simulink model "MPC_Validation"  (R2020a)
settings: Solver=FixedStepAuto  StartTime=0.0  StopTime=tsim  FixedStep=baseRate  RelTol=1e-3  EnableMultiTasking=on
values from neighbouring files (symbols this model uses):
  Ad = -C(7:12,4:9)    [theFastMPCSolver3.m]    (also in theInitializer.m = dss.A)
  ALGORITHM = 5    [Run_Initializer.m]
  baseRate = 0.05    [Run_Initializer.m]
  cdockdeltax = rc+rt-2*dockoffset    (= 0.165)    [theInitializer.m]
  cdockoa = atan(cdockdeltay/cdockdeltax)    [theInitializer.m]
  Cmat = zeros(6*N,9*N)    [theInitializer.m]
  con0 = [n*N, 2*N, N, N, N]    [Run_Initializer.m]
  drop_states_ARM = [ pi/2, pi/2, 0]    [Run_Initializer.m]
  drop_states_BLACK = rand([1,3])/10+init_states_BLACK    [Run_Initializer.m]
  drop_states_BLUE = rand([1,3])/10+init_states_BLUE    [Run_Initializer.m]
  drop_states_RED = rand([1,3])/10+init_states_RED    [Run_Initializer.m]
  ecoa = pi/2    (= 1.57079632679)    [theInitializer.m]
  F_Black_X_nominal = 0.2196    [Run_Initializer.m]
  F_Black_Y_nominal = 0.2825    [Run_Initializer.m]
  F_Blue_X_nominal = 0.2196    [Run_Initializer.m]
  F_Blue_Y_nominal = 0.2825    [Run_Initializer.m]
  F_red_X_nominal = 0.2196    [Run_Initializer.m]
  F_red_Y_nominal = 0.2825    [Run_Initializer.m]
  F_thrusters_BLACK = [F_Black_X_nominal; F_Black_X_nominal;                             F_Black_Y_nominal; F_Black_Y_nominal; F_Black_X_nominal;                              F_Black_X_nominal; F_Black_Y_nominal; F_Black_Y_nominal]    [Run_Initializer.m]
  F_thrusters_BLUE = [F_Blue_X_nominal; F_Blue_X_nominal;                             F_Blue_Y_nominal; F_Blue_Y_nominal; F_Blue_X_nominal;                              F_Blue_X_nominal; F_Blue_Y_nominal; F_Blue_Y_nominal]    [Run_Initializer.m]
  F_thrusters_RED = [F_red_X_nominal; F_red_X_nominal;                             F_red_Y_nominal; F_red_Y_nominal; F_red_X_nominal;                              F_red_X_nominal; F_red_Y_nominal; F_red_Y_nominal]    [Run_Initializer.m]
  Fmat = reshape(repmat([umax,umax,taumax],N,1),3*N,1)    [theInitializer.m]
  gamma = 0.95    [theInitializer.m]
  Gamma1 = 0.0025    [Run_Initializer.m]
  Gamma2 = 100    [Run_Initializer.m]
  Gamma3 = 10    [Run_Initializer.m]
  Gamma4 = 0.001    [Run_Initializer.m]
  Gamma5 = 100    [Run_Initializer.m]
  Gamma6 = 0.001    [Run_Initializer.m]
  H = blkdiag(pattern{:})    [theInitializer.m]
  home_states_BLACK = [ xLength/2, yLength/2, 0]    [Run_Initializer.m]
  home_states_BLUE = [ xLength/2-0.9, yLength/2+0.5, 0]    [Run_Initializer.m]
  home_states_RED = [ xLength/2+0.7, yLength/2, pi]    [Run_Initializer.m]
  init_states_BLACK = [ct;thetat0].'    [Run_Initializer.m]
  init_states_BLUE = [pobj1;0].'    [Run_Initializer.m]
  init_states_RED = xi(1:3).'    [Run_Initializer.m]
  isCONTROL = 0    [Run_Initializer.m]
  Kd_elarm = 0.05    [Run_Initializer.m]
  Kd_sharm = 0.05    [Run_Initializer.m]
  Kd_tb = 0.4    [Run_Initializer.m]
  Kd_tblue = 0.4    [Run_Initializer.m]
  Kd_tr = 0.4    [Run_Initializer.m]
  Kd_wrarm = 0.005    [Run_Initializer.m]
  Kd_xb = 8    [Run_Initializer.m]
  Kd_xblue = 8    [Run_Initializer.m]
  Kd_xr = 8    [Run_Initializer.m]
  Kd_yb = 8    [Run_Initializer.m]
  Kd_yblue = 8    [Run_Initializer.m]
  Kd_yr = 8    [Run_Initializer.m]
  KOZ_actual = KOZ + rc*sqrt(2)*1.1    [theInitializer.m]
  Kp = [0.08 0 0 ... (first row only)    [Run_Initializer.m]
  Kp_elarm = 0.08    [Run_Initializer.m]
  Kp_sharm = 0.15    [Run_Initializer.m]
  Kp_tb = 0.1    [Run_Initializer.m]
  Kp_tblue = 0.1    [Run_Initializer.m]
  Kp_tr = 0.1    [Run_Initializer.m]
  Kp_wrarm = 0.007    [Run_Initializer.m]
  Kp_xb = 2    [Run_Initializer.m]
  Kp_xblue = 2    [Run_Initializer.m]
  Kp_xr = 2    [Run_Initializer.m]
  Kp_yb = 2    [Run_Initializer.m]
  Kp_yblue = 2    [Run_Initializer.m]
  Kp_yr = 2    [Run_Initializer.m]
  Kv = [0.05 0 0 ... (first row only)    [Run_Initializer.m]
  maxiterations = 10    [Run_Initializer.m]
  N = 15    [Run_Initializer.m]    (also in theFastMPCSolver2.m = length(z)/9; theFastMPCSolver3.m = length(z)/9)
  n = size(b,1)    [my_fbsubstitution.m]    (also in theFastMPCSolver3.m)
  noise_variance_BLACK = 0    [Run_Initializer.m]
  noise_variance_BLUE = 0    [Run_Initializer.m]
  noise_variance_RED = 0    [Run_Initializer.m]
  noisemean = 0.1    [Run_Initializer.m]
  pdockoa = atan(rt/cdockdeltax)    [theInitializer.m]
  pdockr = sqrt(cdockdeltax*cdockdeltax + rt*rt)    [theInitializer.m]
  Phase0_End = Phase0_Duration    (= 5)    [Run_Initializer.m]
  Phase1_End = Phase0_Duration + Phase1_Duration    (= 10)    [Run_Initializer.m]
  Phase2_End = Phase0_Duration + Phase1_Duration +                                   Phase2_Duration    (= 36)    [Run_Initializer.m]
  Phase3_End = Phase0_Duration + Phase1_Duration +                                   Phase2_Duration + Phase3_Duration    (= 166)    [Run_Initializer.m]
  Phase3_SubPhase1_End = Phase2_End + Phase3_SubPhase1_Duration    (= 40)    [Run_Initializer.m]
  Phase3_SubPhase2_End = Phase2_End + Phase3_SubPhase1_Duration +                                   Phase3_SubPhase2_Duration    (= 42)    [Run_Initializer.m]
  Phase3_SubPhase3_End = Phase2_End + Phase3_SubPhase1_Duration +                                   Phase3_SubPhase2_Duration +                                  Phase3_SubPhase3_Duration    (= 44)    [Run_Initializer.m]
  Phase3_SubPhase4_End = Phase2_End + Phase3_SubPhase1_Duration +                                   Phase3_SubPhase2_Duration +                                  Phase3_SubPhase3_Duration +                                  Phase3_SubPhase4_Duration    [Run_Initializer.m]
  Phase4_End = Phase0_Duration + Phase1_Duration +                                   Phase2_Duration + Phase3_Duration +                                   Phase4_Duration    (= 186)    [Run_Initializer.m]
  Phase5_End = Phase0_Duration + Phase1_Duration +                                   Phase2_Duration + Phase3_Duration +                                   Phase4_Duration + Phase5_Duration    (= 191)    [Run_Initializer.m]
  rcone = 0.75    [theInitializer.m]
  rdock = sqrt(cdockdeltax*cdockdeltax + cdockdeltay*cdockdeltay)    [theInitializer.m]
  serverRate = 0.1    [Run_Initializer.m]
  Sj = [KOZ_actual^(-2),0; 0,KOZ_actual^(-2)]    [theInitializer.m]
  taumax = umax*rc    (= 0.0225)    [theInitializer.m]
  Td = 2    [Run_Initializer.m]
  thetah = 20.0 * d2r    (= 0.349065850399)    [theInitializer.m]
  thetat_dot = 0 * d2r    (= 0)    [Run_Initializer.m]
  thruster_dist2CG_BLACK = [83.42;-52.58;55.94;-60.05;54.08;-53.92;77.06;-55.94]    [Run_Initializer.m]
  thruster_dist2CG_BLUE = [73.54;-64.46;81.39;-60.11;64.46;-65.94;54.61;-74.39]    [Run_Initializer.m]
  thruster_dist2CG_RED = [49.92;-78.08;70.46;-63.54;81.08;-50.42;57.44;-75.96]    [Run_Initializer.m]
  tol = 0.00015    [Run_Initializer.m]
  Tz_lim_elarm = .1    (= 0.1)    [Run_Initializer.m]
  Tz_lim_sharm = .1    (= 0.1)    [Run_Initializer.m]
  Tz_lim_wrarm = .1    (= 0.1)    [Run_Initializer.m]
  Umat = zeros(3*N,9*N)    [theInitializer.m]
  umax = 0.15    [theInitializer.m]
  vobj1 = [0.00;0.00]    [Run_Initializer.m]
  vtar = [0.0;0.0]    [Run_Initializer.m]
undefined symbols (not defined in the file or in its folder): DiscIntNeverNeededParam, model_param, platformSelection, simMode, WhoAmI
libraries: dspstat3 x23, dspsigops x15, embdlinuxlib x10, raspberrypiBasiclib x10, simulink x8, MainLibrary x7, mspfiltlib x3, dsparch4 x3, dspswit3 x2, sensehatlib x1
(part 4 of 18)

== system MPC_Validation/Phase #5: Hold Home/Change BLUE Behavior ==
  note: PD Control Law - WHITE
  note: Additional blocks are stored here.
  note: A simple PD control law is used here to command the platform to it's initial position, as defined in the initializer.
  note: Additional Blocks
  Action Port : ActionPort  ActionPortLabel=if(u1 == 3 | u2 == 1)
  BLUE_Fx : DataStoreWrite  DataStoreName=BLUE_Fx
  BLUE_Fy : DataStoreWrite  DataStoreName=BLUE_Fy
  BLUE_Px : DataStoreRead  DataStoreName=BLUE_Px
  "BLUE_Py " : DataStoreRead  DataStoreName=BLUE_Py
  BLUE_Rz : DataStoreRead  DataStoreName=BLUE_Rz
  BLUE_Tz : DataStoreWrite  DataStoreName=BLUE_Tz
  Custom Discrete PD (Attitude) : Subsystem
  Custom Discrete PD (X-Position) : Subsystem
  Custom Discrete PD (Y-Position) : Subsystem
  Data Store Write3 : DataStoreWrite  DataStoreName=Float_State
  Desired Attitude (BLUE) : Constant  Value=home_states_BLUE(3)  SampleTime=-1
  Desired Px (BLUE) : Constant  Value=home_states_BLUE(1)  SampleTime=-1
  Desired Py (BLUE) : Constant  Value=home_states_BLUE(2)  SampleTime=-1
  Hough Control : Subsystem
  Puck State : Constant
  Subtract : Sum  Inputs=+-
  Subtract1 : Sum  Inputs=+-
  wires:
  Puck State/1 -> Data Store Write3/1
  Custom Discrete PD (Y-Position)/1(Fy) -> BLUE_Fy/1
  Custom Discrete PD (X-Position)/1(Fx) -> BLUE_Fx/1
  Subtract1/1 -> Custom Discrete PD (Y-Position)/1(ey)
  "BLUE_Py "/1 -> Subtract1/2
  Desired Px (BLUE)/1 -> Subtract/1
  Hough Control/1(Err) -> Custom Discrete PD (Attitude)/1(ez)
  Subtract/1 -> Custom Discrete PD (X-Position)/1(ex)
  Custom Discrete PD (Attitude)/1(Tz) -> BLUE_Tz/1
  BLUE_Rz/1 -> Hough Control/2(Act)
  Desired Py (BLUE)/1 -> Subtract1/1
  BLUE_Px/1 -> Subtract/2
  Desired Attitude (BLUE)/1 -> Hough Control/1(Ref)

== system MPC_Validation/Phase #5: Hold Home/Change RED Behavior ==
  note: PD Control Law - RED
  note: Additional Blocks
  note: Additional blocks are stored above. Note that to control attitude using the RW, simply replace RED_Tz with RED_Tz_RW.
  note: A simple PD control law is used here to command the platform to it's home position, as defined in the initializer.
  note: ARM Control Law - RED
  Action Port : ActionPort  ActionPortLabel=if(u1 == 1 | u2 == 1)
  Constant1 : Constant  Value=0
  Constant3 : Constant  Value=platformSelection
  Custom Discrete PD (Attitude) : Subsystem
  Custom Discrete PD (X-Position) : Subsystem
  Custom Discrete PD (Y-Position) : Subsystem
  Data Store Write1 : DataStoreWrite  DataStoreName=MPC_State
  Data Store Write3 : DataStoreWrite  DataStoreName=Float_State
  Data Store Write4 : DataStoreWrite  DataStoreName=MPC_State
  Desired Px (BLACK) : Constant  Value=home_states_RED(1)  SampleTime=-1
  Desired Px (BLACK)1 : Constant  Value=home_states_RED(2)  SampleTime=-1
  Desired Px (BLACK)2 : Constant  Value=home_states_RED(3)  SampleTime=-1
  Hough Control : Subsystem
  If : If  IfExpression=u1 == 4 | u1 == 5 | u1 == 10 | u1 == 11
  MPC State : Constant  Value=0
  MPC State1 : Constant  Value=0
  Puck State : Constant
  RED : Subsystem  TreatAsAtomicUnit=on
  RED+ARM : Subsystem  TreatAsAtomicUnit=on
  RED_Fx : DataStoreWrite  DataStoreName=RED_Fx
  RED_Fy : DataStoreWrite  DataStoreName=RED_Fy
  RED_Px : DataStoreRead  DataStoreName=RED_Px
  "RED_Py " : DataStoreRead  DataStoreName=RED_Py
  RED_Rz : DataStoreRead  DataStoreName=RED_Rz
  RED_Tz : DataStoreWrite  DataStoreName=RED_Tz
  RED_Tz_RW : DataStoreWrite  DataStoreName=RED_Tz_RW
  Subtract : Sum  Inputs=+-
  Subtract1 : Sum  Inputs=+-
  wires:
  Constant1/1 -> RED_Tz_RW/1
  Puck State/1 -> Data Store Write3/1
  Desired Px (BLACK)1/1 -> Subtract1/1
  Custom Discrete PD (Attitude)/1(Tz) -> RED_Tz/1
  "RED_Py "/1 -> Subtract1/2
  RED_Rz/1 -> Hough Control/2(Act)
  Desired Px (BLACK)/1 -> Subtract/1
  Custom Discrete PD (Y-Position)/1(Fy) -> RED_Fy/1
  Subtract1/1 -> Custom Discrete PD (Y-Position)/1(ey)
  Custom Discrete PD (X-Position)/1(Fx) -> RED_Fx/1
  Subtract/1 -> Custom Discrete PD (X-Position)/1(ex)
  Hough Control/1(Err) -> Custom Discrete PD (Attitude)/1(ez)
  Desired Px (BLACK)2/1 -> Hough Control/1(Ref)
  RED_Px/1 -> Subtract/2
  If/1 -> RED+ARM/Action
  If/2 -> RED/Action
  Constant3/1 -> If/1
  MPC State/1 -> Data Store Write4/1
  MPC State1/1 -> Data Store Write1/1

== system MPC_Validation/Phase #5: Hold Home/Is this a simulation? ==
  Constant : Constant  Value=simMode  SampleTime=-1
  isSim : Outport  VectorParamsAs1DForOutWhenUnconnected=off
  wires:
  Constant/1 -> isSim/1

== system MPC_Validation/Phase #6: Stop Floating and Spin Down RW/Change BLACK Behavior ==
  note: At the end of the experiment, the pucks must be turned off.
  note: At the end of the experiment, all thrust and arms movement must cease.
  Action Port : ActionPort  ActionPortLabel=if(u1 == 2 | u2 == 1)
  BLACK_Fx : DataStoreWrite  DataStoreName=BLACK_Fx
  BLACK_Fy : DataStoreWrite  DataStoreName=BLACK_Fy
  BLACK_Tz : DataStoreWrite  DataStoreName=BLACK_Tz
  Constant3 : Constant  Value=0
  Constant4 : Constant  Value=0
  Constant5 : Constant  Value=0
  Data Store Write3 : DataStoreWrite  DataStoreName=Float_State
  Puck State : Constant  Value=0
  wires:
  Constant3/1 -> BLACK_Fx/1
  Constant5/1 -> BLACK_Tz/1
  Constant4/1 -> BLACK_Fy/1
  Puck State/1 -> Data Store Write3/1

== system MPC_Validation/Phase #6: Stop Floating and Spin Down RW/Change BLUE Behavior ==
  note: Before getting good data, the platforms must NOT be floating. So, float is set to be "off".
  note: For the initialization phase, we do not want any thrust. Thus, all commanded forces are zero.
  Action Port : ActionPort  ActionPortLabel=if(u1 == 3 | u2 == 1)
  BLUE_Fx : DataStoreWrite  DataStoreName=BLUE_Fx
  BLUE_Fy : DataStoreWrite  DataStoreName=BLUE_Fy
  BLUE_Tz : DataStoreWrite  DataStoreName=BLUE_Tz
  Constant3 : Constant  Value=0
  Constant4 : Constant  Value=0
  Constant5 : Constant  Value=0
  Data Store Write4 : DataStoreWrite  DataStoreName=Float_State
  Puck State : Constant  Value=0
  wires:
  Constant3/1 -> BLUE_Fx/1
  Constant5/1 -> BLUE_Tz/1
  Constant4/1 -> BLUE_Fy/1
  Puck State/1 -> Data Store Write4/1

== system MPC_Validation/Phase #6: Stop Floating and Spin Down RW/Change RED Behavior ==
  note: At the end of the experiment, the pucks must be turned off.
  note: At the end of the experiment, all thrust and arms movement must cease.
  note: Once the platform has settled, the RW must be slowly desaturated (assuming it has been used).
  Action Port : ActionPort  ActionPortLabel=if(u1 == 1 | u2 == 1)
  Constant{,1..2,4..6} (6 alike) : Constant  Value=0
  Data Store Write : DataStoreWrite  DataStoreName=RED_Tz_Shoulder
  Data Store Write1 : DataStoreWrite  DataStoreName=RED_Tz_Elbow
  Data Store Write2 : DataStoreWrite  DataStoreName=RED_Tz_Wrist
  Data Store Write3 : DataStoreWrite  DataStoreName=Float_State
  Data Store Write4 : DataStoreWrite  DataStoreName=MPC_State
  Gain : Gain  Gain=-1
  MPC State : Constant  Value=0
  Puck State : Constant  Value=0
  RED_Fx : DataStoreWrite  DataStoreName=RED_Fx
  RED_Fy : DataStoreWrite  DataStoreName=RED_Fy
  RED_Tz : DataStoreWrite  DataStoreName=RED_Tz
  RED_Tz_RW : DataStoreWrite  DataStoreName=RED_Tz_RW
  RED_dRz_Speed : DataStoreRead  DataStoreName=RED_dRz_RW_Sat
  Saturation : Saturate  UpperLimit=0.005  LowerLimit=-0.005
  wires:
  Constant/1 -> RED_Fx/1
  Constant6/1 -> Data Store Write2/1
  Constant5/1 -> Data Store Write1/1
  RED_dRz_Speed/1 -> Gain/1
  Constant4/1 -> Data Store Write/1
  Saturation/1 -> RED_Tz_RW/1
  Constant1/1 -> RED_Fy/1
  Gain/1 -> Saturation/1
  Constant2/1 -> RED_Tz/1
  Puck State/1 -> Data Store Write3/1
  MPC State/1 -> Data Store Write4/1

== system MPC_Validation/Phase #6: Stop Floating and Spin Down RW/Is this a simulation? ==
  Constant : Constant  Value=simMode  SampleTime=-1
  isSim : Outport  VectorParamsAs1DForOutWhenUnconnected=off
  wires:
  Constant/1 -> isSim/1

== system MPC_Validation/Simulate Plant Dynamics/BLACK Dynamics ==
  note: Above is the dynamic model for the BLACK platform.
  BLACK Dynamics Model : Subsystem  SystemSampleTime=serverRate
  BLACK_Fx_Sat : DataStoreRead  DataStoreName=BLACK_Fx_Sat
  BLACK_Fy_Sat : DataStoreRead  DataStoreName=BLACK_Fy_Sat
  BLACK_IMU_Ax_I : DataStoreWrite  DataStoreName=BLACK_IMU_Ax_I
  BLACK_IMU_Ay_I : DataStoreWrite  DataStoreName=BLACK_IMU_Ay_I
  BLACK_IMU_R : DataStoreWrite  DataStoreName=BLACK_IMU_R
  BLACK_Px : DataStoreWrite  DataStoreName=BLACK_Px
  BLACK_Py : DataStoreWrite  DataStoreName=BLACK_Py
  BLACK_Rz : DataStoreWrite  DataStoreName=BLACK_Rz
  BLACK_RzD : DataStoreWrite  DataStoreName=BLACK_RzD
  BLACK_Tz_Sat : DataStoreRead  DataStoreName=BLACK_Tz_Sat
  BLACK_Vx : DataStoreWrite  DataStoreName=BLACK_Vx
  BLACK_Vy : DataStoreWrite  DataStoreName=BLACK_Vy
  Demux1 : Demux  Outputs=3
  Demux2 : Demux  Outputs=3
  Mux1 : Mux  Inputs=3
  Random Number : RandomNumber  Mean=noisemean  Variance=1.5e-6
  Random Number1 : RandomNumber  Mean=noisemean  Variance=1.5e-6
  Random Number2 : RandomNumber  Mean=noisemean  Variance=1.5e-6
  Sample and Hold Data to Match PhaseSpace (BLACK) : Subsystem
  Sum1 : Sum  Inputs=|++
  Sum2 : Sum  Inputs=|++
  Sum3 : Sum  Inputs=|++
  "x_dot -> x13" : Subsystem
  "x_dot -> x14" : Subsystem
  "x_dot -> x4" : Subsystem
  "x_dot -> x5" : Subsystem
  "x_dot -> x6" : Subsystem
  wires:
  BLACK_Fy_Sat/1 -> Mux1/2
  BLACK_Tz_Sat/1 -> Mux1/3
  Demux1/1 -> BLACK_Px/1
  "x_dot -> x4"/1(dy(t)/dt) -> "x_dot -> x13"/1(y(t)), BLACK_Vx/1
  "x_dot -> x6"/1(dy(t)/dt) -> Sum3/1, BLACK_RzD/1
  Demux1/2 -> BLACK_Py/1
  "x_dot -> x5"/1(dy(t)/dt) -> "x_dot -> x14"/1(y(t)), BLACK_Vy/1
  BLACK_Fx_Sat/1 -> Mux1/1
  Demux2/2 -> "x_dot -> x5"/1(y(t))
  Mux1/1 -> BLACK Dynamics Model/1(control_inputs)
  Demux2/3 -> "x_dot -> x6"/1(y(t))
  Demux1/3 -> BLACK_Rz/1
  Sum3/1 -> BLACK_IMU_R/1
  BLACK Dynamics Model/1(states) -> Sample and Hold Data to Match PhaseSpace (BLACK)/1(states)
  Demux2/1 -> "x_dot -> x4"/1(y(t))
  Sample and Hold Data to Match PhaseSpace (BLACK)/1(states_hold) -> Demux2/1, Demux1/1
  Sum1/1 -> BLACK_IMU_Ax_I/1
  "x_dot -> x13"/1(dy(t)/dt) -> Sum1/1
  Sum2/1 -> BLACK_IMU_Ay_I/1
  Random Number/1 -> Sum2/2
  Random Number2/1 -> Sum3/2
  Random Number1/1 -> Sum1/2
  "x_dot -> x14"/1(dy(t)/dt) -> Sum2/1

== system MPC_Validation/Simulate Plant Dynamics/BLUE Dynamics ==
  note: Above is the dynamic model for the BLUE platform.
  BLUE  Dynamics Model : Subsystem  SystemSampleTime=serverRate
  "BLUE_Fx_Sat " : DataStoreRead  DataStoreName=BLUE_Fx_Sat
  BLUE_Fy_Sat : DataStoreRead  DataStoreName=BLUE_Fy_Sat
  BLUE_IMU_Ax_I : DataStoreWrite  DataStoreName=BLUE_IMU_Ax_I
  BLUE_IMU_Ay_I : DataStoreWrite  DataStoreName=BLUE_IMU_Ay_I
  BLUE_IMU_R : DataStoreWrite  DataStoreName=BLUE_IMU_R
  "BLUE_Px " : DataStoreWrite  DataStoreName=BLUE_Px
  BLUE_Py : DataStoreWrite  DataStoreName=BLUE_Py
  BLUE_Rz : DataStoreWrite  DataStoreName=BLUE_Rz
  BLUE_RzD : DataStoreWrite  DataStoreName=BLUE_RzD
  BLUE_Tz_Sat : DataStoreRead  DataStoreName=BLUE_Tz_Sat
  BLUE_Vx : DataStoreWrite  DataStoreName=BLUE_Vx
  BLUE_Vy : DataStoreWrite  DataStoreName=BLUE_Vy
  Demux4 : Demux  Outputs=3
  Demux5 : Demux  Outputs=3
  Mux2 : Mux  Inputs=3
  Random Number3 : RandomNumber  Mean=noisemean  Variance=1.5e-6
  Random Number4 : RandomNumber  Mean=noisemean  Variance=1.5e-6
  Random Number5 : RandomNumber  Variance=1.5e-6
  Sample and Hold Data to Match PhaseSpace (BLUE) : Subsystem
  Sum4 : Sum  Inputs=|++
  Sum5 : Sum  Inputs=|++
  Sum6 : Sum  Inputs=|++
  "x_dot -> x16" : Subsystem
  "x_dot -> x17" : Subsystem
  "x_dot -> x7" : Subsystem
  "x_dot -> x8" : Subsystem
  "x_dot -> x9" : Subsystem
  wires:
  Sample and Hold Data to Match PhaseSpace (BLUE)/1(states_hold) -> Demux5/1, Demux4/1
  Demux5/3 -> "x_dot -> x9"/1(y(t))
  Demux4/1 -> "BLUE_Px "/1
  Demux4/2 -> BLUE_Py/1
  "BLUE_Fx_Sat "/1 -> Mux2/1
  BLUE_Fy_Sat/1 -> Mux2/2
  Demux5/1 -> "x_dot -> x7"/1(y(t))
  BLUE_Tz_Sat/1 -> Mux2/3
  Demux4/3 -> BLUE_Rz/1
  BLUE  Dynamics Model/1(states) -> Sample and Hold Data to Match PhaseSpace (BLUE)/1(states)
  "x_dot -> x8"/1(dy(t)/dt) -> BLUE_Vy/1, "x_dot -> x17"/1(y(t))
  Mux2/1 -> BLUE  Dynamics Model/1(control_inputs)
  "x_dot -> x7"/1(dy(t)/dt) -> "x_dot -> x16"/1(y(t)), BLUE_Vx/1
  Sum5/1 -> BLUE_IMU_Ay_I/1
  "x_dot -> x9"/1(dy(t)/dt) -> Sum6/1, BLUE_RzD/1
  Sum4/1 -> BLUE_IMU_Ax_I/1
  Demux5/2 -> "x_dot -> x8"/1(y(t))
  Random Number3/1 -> Sum5/2
  "x_dot -> x16"/1(dy(t)/dt) -> Sum4/1
  "x_dot -> x17"/1(dy(t)/dt) -> Sum5/1
  Random Number4/1 -> Sum4/2
  Sum6/1 -> BLUE_IMU_R/1
  Random Number5/1 -> Sum6/2

== system MPC_Validation/Simulate Plant Dynamics/IMU Model ==
  Compare To Zero : simulink/Logic and Bit Operations/Compare To Zero  relop===  OutDataTypeStr=boolean
  Compare To Zero1 : simulink/Logic and Bit Operations/Compare To Zero  relop===  OutDataTypeStr=boolean
  Compare To Zero2 : simulink/Logic and Bit Operations/Compare To Zero  relop===  OutDataTypeStr=boolean
  Data Store Read1 : DataStoreRead  DataStoreName=BLUE_Rz
  Data Store Read2 : DataStoreRead  DataStoreName=BLACK_Rz
  Data Store Read3 : DataStoreRead  DataStoreName=BLUE_IMU_R
  Data Store Read4 : DataStoreRead  DataStoreName=BLACK_IMU_R
  Data Store Read5 : DataStoreRead  DataStoreName=RED_Rz
  Data Store Read6 : DataStoreRead  DataStoreName=RED_IMU_R
  Discrete-Time Integrator : DiscreteIntegrator  IntegratorMethod=Integration: Backward Euler  ExternalReset=either  InitialConditionSource=external  SampleTime=-1  ICPrevOutput=DiscIntNeverNeededParam  ICPrevScaledInput=DiscIntNeverNeededParam
  Discrete-Time Integrator1 : DiscreteIntegrator  IntegratorMethod=Integration: Backward Euler  ExternalReset=either  InitialConditionSource=external  SampleTime=-1  ICPrevOutput=DiscIntNeverNeededParam  ICPrevScaledInput=DiscIntNeverNeededParam
  Discrete-Time Integrator2 : DiscreteIntegrator  IntegratorMethod=Integration: Backward Euler  ExternalReset=either  InitialConditionSource=external  SampleTime=-1  ICPrevOutput=DiscIntNeverNeededParam  ICPrevScaledInput=DiscIntNeverNeededParam
  RED_Px1 : DataStoreWrite  DataStoreName=BLACK_IMU_Psi
  RED_Px2 : DataStoreWrite  DataStoreName=RED_IMU_Psi
  RED_Px4 : DataStoreWrite  DataStoreName=BLUE_IMU_Psi
  wires:
  Data Store Read5/1 -> Compare To Zero2/1, Discrete-Time Integrator2/3
  Data Store Read1/1 -> Compare To Zero/1, Discrete-Time Integrator/3
  Discrete-Time Integrator/1 -> RED_Px4/1
  Data Store Read6/1 -> Discrete-Time Integrator2/1
  Compare To Zero1/1 -> Discrete-Time Integrator1/2
  Data Store Read2/1 -> Compare To Zero1/1, Discrete-Time Integrator1/3
  Data Store Read4/1 -> Discrete-Time Integrator1/1
  Compare To Zero/1 -> Discrete-Time Integrator/2
  Data Store Read3/1 -> Discrete-Time Integrator/1
  Discrete-Time Integrator2/1 -> RED_Px2/1
  Discrete-Time Integrator1/1 -> RED_Px1/1
  Compare To Zero2/1 -> Discrete-Time Integrator2/2

== system MPC_Validation/Simulate Plant Dynamics/RED and ARM Dynamics ==
  Constant : Constant  Value=platformSelection
  If : If  IfExpression=u1 == 4 | u1 == 5 | u1 == 10 | u1 == 11
  RED + ARM : Subsystem  TreatAsAtomicUnit=on
  RED Only : Subsystem  TreatAsAtomicUnit=on
  wires:
  If/1 -> RED + ARM/Action
  Constant/1 -> If/1
  If/2 -> RED Only/Action

== system MPC_Validation/Subsystem1/If Action Subsystem ==
  Action Port : ActionPort  ActionPortLabel=if(u1 == u2)
  Constant : Constant
  Data Store Read : DataStoreRead  DataStoreName=TRIGGER
  Data Store Write : DataStoreWrite  DataStoreName=COUNTER
  Data Store Write1 : DataStoreWrite  DataStoreName=TRIGGER
  If : If  IfExpression=u1 > 0.5
  If Action Subsystem : Subsystem  TreatAsAtomicUnit=on
  If Action Subsystem1 : Subsystem  TreatAsAtomicUnit=on
  Merge : Merge
  wires:
  Constant/1 -> Data Store Write/1
  Data Store Read/1 -> If/1
  If/1 -> If Action Subsystem/Action
  If/2 -> If Action Subsystem1/Action
  If Action Subsystem/1(Out1) -> Merge/1
  If Action Subsystem1/1(Out1) -> Merge/2
  Merge/1 -> Data Store Write1/1

== system MPC_Validation/Subsystem1/If Action Subsystem1 ==
  Action Port : ActionPort  ActionPortLabel=else
  Constant7 : Constant
  Data Store Read1 : DataStoreRead  DataStoreName=COUNTER
  Data Store Write : DataStoreWrite  DataStoreName=COUNTER
  Sum : Sum  Inputs=|++
  wires:
  Constant7/1 -> Sum/2
  Data Store Read1/1 -> Sum/1
  Sum/1 -> Data Store Write/1

== system MPC_Validation/Subsystem1/If Action Subsystem2 ==
  Action Port : ActionPort  ActionPortLabel=if(u1 > 0)
  Data Store Read : DataStoreRead  DataStoreName=TRIGGER
  Out1 : Outport
  wires:
  Data Store Read/1 -> Out1/1

== system MPC_Validation/Subsystem1/If Action Subsystem3 ==
  Action Port : ActionPort  ActionPortLabel=else
  Constant : Constant  Value=0
  Out1 : Outport
  wires:
  Constant/1 -> Out1/1

== system MPC_Validation/Triggered Subsystem/Desired x-pos ==
  Constant : Constant  Value=vobj1
  Constant1 : Constant  Value=Phase3_SubPhase3_End
  Constant2 : Constant  Commented=on  Value=Phase1_End
  Demux : Demux  Outputs=2
  Desired Attitude (BLACK) : Constant  Value=init_states_BLUE(1)  SampleTime=-1
  Product : Product
  Sum : Sum  Inputs=+-
  Sum1 : Sum
  Terminator : Terminator
  Universal_Time : DataStoreRead  DataStoreName=Univ_Time
  Ref : Outport
  wires:
  Product/1 -> Sum1/2
  Constant1/1 -> Sum/2
  Sum/1 -> Product/2
  Universal_Time/1 -> Sum/1
  Sum1/1 -> Ref/1
  Desired Attitude (BLACK)/1 -> Sum1/1
  Constant/1 -> Demux/1
  Demux/1 -> Product/1
  Demux/2 -> Terminator/1

== system MPC_Validation/Triggered Subsystem/Desired y-pos ==
  Constant : Constant  Value=vobj1
  Constant1 : Constant  Value=Phase3_SubPhase3_End
  Constant2 : Constant  Commented=on  Value=Phase1_End
  Demux : Demux  Outputs=2
  Desired Attitude (BLACK) : Constant  Value=init_states_BLUE(2)  SampleTime=-1
  Product : Product
  Sum : Sum  Inputs=+-
  Sum1 : Sum
  Terminator : Terminator
  Universal_Time : DataStoreRead  DataStoreName=Univ_Time
  Ref : Outport
  wires:
  Product/1 -> Sum1/2
  Constant1/1 -> Sum/2
  Sum/1 -> Product/2
  Universal_Time/1 -> Sum/1
  Sum1/1 -> Ref/1
  Desired Attitude (BLACK)/1 -> Sum1/1
  Constant/1 -> Demux/1
  Demux/1 -> Terminator/1
  Demux/2 -> Product/1

== system MPC_Validation/Triggered Subsystem/If Action Subsystem ==
  Action Port : ActionPort  ActionPortLabel=if(u1 == 5 & u2 == 0)
  Data Store Read : DataStoreRead  DataStoreName=RED_RzD
  Data Store Read1 : DataStoreRead  DataStoreName=RED_Vy
  Data Store Read10 : DataStoreRead  DataStoreName=BLUE_Px
  Data Store Read11 : DataStoreRead  DataStoreName=BLUE_Py
  Data Store Read12 : DataStoreRead  DataStoreName=BLACK_Vx_MF
  Data Store Read14 : DataStoreRead  DataStoreName=BLUE_Vx_MF
  Data Store Read15 : DataStoreRead  DataStoreName=BLUE_Vy_MF
  Data Store Read16 : DataStoreRead  DataStoreName=BLACK_Rz
  Data Store Read17 : DataStoreRead  DataStoreName=BLACK_RzD_MF
  Data Store Read18 : DataStoreRead  DataStoreName=BLACK_Vy_MF
  Data Store Read2 : DataStoreRead  DataStoreName=RED_Vx
  Data Store Read3 : DataStoreRead  DataStoreName=RED_Rz
  Data Store Read4 : DataStoreRead  DataStoreName=RED_Py
  Data Store Read5 : DataStoreRead  DataStoreName=RED_Px
  Data Store Read6 : DataStoreRead  DataStoreName=X0
  Data Store Read7 : DataStoreRead  DataStoreName=RHOLD
  Data Store Read8 : DataStoreRead  DataStoreName=BLACK_Px
  Data Store Read9 : DataStoreRead  DataStoreName=BLACK_Py
  Data Store Write : DataStoreWrite  DataStoreName=CPUTIME
  Data Store Write4 : DataStoreWrite  DataStoreName=X0
  Data Store Write5 : DataStoreWrite  DataStoreName=RHOLD
  Demux : Demux  Outputs=3
  MPC : MATLAB Function  TreatAsAtomicUnit=on
  Mux : Mux  Inputs=6
  Mux{1..4} (4 alike) : Mux  Inputs=2
  RED_Fx : DataStoreWrite  DataStoreName=RED_Fx
  RED_Fy : DataStoreWrite  DataStoreName=RED_Fy
  RED_Tz : DataStoreWrite  DataStoreName=RED_Tz
  Scope : Scope
  Scope1 : Scope
  wires:
  MPC/4(CPUTIME) -> Data Store Write/1
  Data Store Read10/1 -> Mux2/1
  Data Store Read4/1 -> Mux/2
  Data Store Read8/1 -> Mux1/1
  Data Store Read5/1 -> Mux/1
  Data Store Read11/1 -> Mux2/2
  Data Store Read3/1 -> Mux/3
  Mux/1 -> MPC/1(xi)
  Demux/3 -> RED_Tz/1
  Demux/1 -> RED_Fx/1
  MPC/1(CONTROL) -> Demux/1, Scope/1
  Demux/2 -> RED_Fy/1
  MPC/3(rhold) -> Scope1/1, Data Store Write5/1
  MPC/2(x0) -> Data Store Write4/1
  Data Store Read9/1 -> Mux1/2
  Mux3/1 -> MPC/6(vtar)
  Mux2/1 -> MPC/5(pobj1)
  Data Store Read7/1 -> MPC/3("rhold ")
  Data Store Read6/1 -> MPC/2("x0 ")
  Mux4/1 -> MPC/7(vobj1)
  Data Store Read16/1 -> MPC/8(thetat0)
  Mux1/1 -> MPC/4(ct)
  Data Store Read2/1 -> Mux/4
  Data Store Read1/1 -> Mux/5
  Data Store Read/1 -> Mux/6
  Data Store Read14/1 -> Mux4/1
  Data Store Read15/1 -> Mux4/2
  Data Store Read18/1 -> Mux3/2
  Data Store Read17/1 -> MPC/9(thetat_dot)
  Data Store Read12/1 -> Mux3/1

== system MPC_Validation/Triggered Subsystem/If Action Subsystem1 ==
  Action Port : ActionPort  ActionPortLabel=elseif( u1 == 6 & u2 == 0)
  Data Store Read : DataStoreRead  DataStoreName=RED_RzD
  Data Store Read1 : DataStoreRead  DataStoreName=RED_Vy
  Data Store Read10 : DataStoreRead  DataStoreName=BLUE_Px
  Data Store Read11 : DataStoreRead  DataStoreName=BLUE_Py
  Data Store Read12 : DataStoreRead  DataStoreName=BLACK_Vx
  Data Store Read13 : DataStoreRead  DataStoreName=BLACK_Vy
  Data Store Read14 : DataStoreRead  DataStoreName=BLUE_Vx
  Data Store Read15 : DataStoreRead  DataStoreName=BLUE_Vy
  Data Store Read16 : DataStoreRead  DataStoreName=BLACK_Rz
  Data Store Read17 : DataStoreRead  DataStoreName=BLACK_RzD
  Data Store Read2 : DataStoreRead  DataStoreName=RED_Vx
  Data Store Read3 : DataStoreRead  DataStoreName=RED_Rz
  Data Store Read4 : DataStoreRead  DataStoreName=RED_Py
  Data Store Read5 : DataStoreRead  DataStoreName=RED_Px
  Data Store Read6 : DataStoreRead  DataStoreName=X0
  Data Store Read7 : DataStoreRead  DataStoreName=RHOLD
  Data Store Read8 : DataStoreRead  DataStoreName=BLACK_Px
  Data Store Read9 : DataStoreRead  DataStoreName=BLACK_Py
  Data Store Write : DataStoreWrite  DataStoreName=CPUTIME
  Data Store Write4 : DataStoreWrite  DataStoreName=X0
  Data Store Write5 : DataStoreWrite  DataStoreName=RHOLD
  Demux : Demux  Outputs=3
  MPC : MATLAB Function  TreatAsAtomicUnit=on
  Mux : Mux  Inputs=6
  Mux{1..4} (4 alike) : Mux  Inputs=2
  RED_Fx : DataStoreWrite  DataStoreName=RED_Fx
  RED_Fy : DataStoreWrite  DataStoreName=RED_Fy
  RED_Tz : DataStoreWrite  DataStoreName=RED_Tz
  Scope : Scope
  Scope1 : Scope
  wires:
  MPC/4(CPUTIME) -> Data Store Write/1
  Data Store Read10/1 -> Mux2/1
  Data Store Read4/1 -> Mux/2
  Data Store Read14/1 -> Mux4/1
  Data Store Read8/1 -> Mux1/1
  Data Store Read5/1 -> Mux/1
  Data Store Read11/1 -> Mux2/2
  Data Store Read3/1 -> Mux/3
  Data Store Read13/1 -> Mux3/2
  Data Store Read1/1 -> Mux/5
  Mux/1 -> MPC/1(xi)
  Demux/3 -> RED_Tz/1
  Demux/1 -> RED_Fx/1
  MPC/1(CONTROL) -> Demux/1, Scope/1
  Data Store Read/1 -> Mux/6
  Demux/2 -> RED_Fy/1
  MPC/3(rhold) -> Scope1/1, Data Store Write5/1
  MPC/2(x0) -> Data Store Write4/1
  Data Store Read15/1 -> Mux4/2
  Data Store Read2/1 -> Mux/4
  Data Store Read9/1 -> Mux1/2
  Mux3/1 -> MPC/6(vtar)
  Data Store Read12/1 -> Mux3/1
  Mux2/1 -> MPC/5(pobj1)
  Data Store Read7/1 -> MPC/3("rhold ")
  Data Store Read6/1 -> MPC/2("x0 ")
  Mux4/1 -> MPC/7(vobj1)
  Data Store Read16/1 -> MPC/8(thetat0)
  Data Store Read17/1 -> MPC/9(thetat_dot)
  Mux1/1 -> MPC/4(ct)

== system MPC_Validation/Triggered Subsystem/If Action Subsystem2 ==
  Action Port : ActionPort  ActionPortLabel=elseif( u1 == 7 & u2 == 0)
  Data Store Read : DataStoreRead  DataStoreName=RED_RzD
  Data Store Read1 : DataStoreRead  DataStoreName=RED_Vy
  Data Store Read10 : DataStoreRead  DataStoreName=BLUE_Px
  Data Store Read11 : DataStoreRead  DataStoreName=BLUE_Py
  Data Store Read12 : DataStoreRead  DataStoreName=BLACK_Vx
  Data Store Read13 : DataStoreRead  DataStoreName=BLACK_Vy
  Data Store Read14 : DataStoreRead  DataStoreName=BLUE_Vx
  Data Store Read15 : DataStoreRead  DataStoreName=BLUE_Vy
  Data Store Read16 : DataStoreRead  DataStoreName=BLACK_Rz
  Data Store Read17 : DataStoreRead  DataStoreName=BLACK_RzD
  Data Store Read2 : DataStoreRead  DataStoreName=RED_Vx
  Data Store Read3 : DataStoreRead  DataStoreName=RED_Rz
  Data Store Read4 : DataStoreRead  DataStoreName=RED_Py
  Data Store Read5 : DataStoreRead  DataStoreName=RED_Px
  Data Store Read6 : DataStoreRead  DataStoreName=X0
  Data Store Read7 : DataStoreRead  DataStoreName=RHOLD
  Data Store Read8 : DataStoreRead  DataStoreName=BLACK_Px
  Data Store Read9 : DataStoreRead  DataStoreName=BLACK_Py
  Data Store Write : DataStoreWrite  DataStoreName=CPUTIME
  Data Store Write4 : DataStoreWrite  DataStoreName=X0
  Data Store Write5 : DataStoreWrite  DataStoreName=RHOLD
  Demux : Demux  Outputs=3
  MPC : MATLAB Function  TreatAsAtomicUnit=on
  Mux : Mux  Inputs=6
  Mux{1..4} (4 alike) : Mux  Inputs=2
  RED_Fx : DataStoreWrite  DataStoreName=RED_Fx
  RED_Fy : DataStoreWrite  DataStoreName=RED_Fy
  RED_Tz : DataStoreWrite  DataStoreName=RED_Tz
  Scope : Scope
  Scope1 : Scope
  wires:
  MPC/4(CPUTIME) -> Data Store Write/1
  Data Store Read10/1 -> Mux2/1
  Data Store Read4/1 -> Mux/2
  Data Store Read14/1 -> Mux4/1
  Data Store Read8/1 -> Mux1/1
  Data Store Read5/1 -> Mux/1
  Data Store Read11/1 -> Mux2/2
  Data Store Read3/1 -> Mux/3
  Data Store Read13/1 -> Mux3/2
  Data Store Read1/1 -> Mux/5
  Mux/1 -> MPC/1(xi)
  Demux/3 -> RED_Tz/1
  Demux/1 -> RED_Fx/1
  MPC/1(CONTROL) -> Demux/1, Scope/1
  Data Store Read/1 -> Mux/6
  Demux/2 -> RED_Fy/1
  MPC/3(rhold) -> Scope1/1, Data Store Write5/1
  MPC/2(x0) -> Data Store Write4/1
  Data Store Read15/1 -> Mux4/2
  Data Store Read2/1 -> Mux/4
  Data Store Read9/1 -> Mux1/2
  Mux3/1 -> MPC/6(vtar)
  Data Store Read12/1 -> Mux3/1
  Mux2/1 -> MPC/5(pobj1)
  Data Store Read7/1 -> MPC/3("rhold ")
  Data Store Read6/1 -> MPC/2("x0 ")
  Mux4/1 -> MPC/7(vobj1)
  Data Store Read16/1 -> MPC/8(thetat0)
  Data Store Read17/1 -> MPC/9(thetat_dot)
  Mux1/1 -> MPC/4(ct)

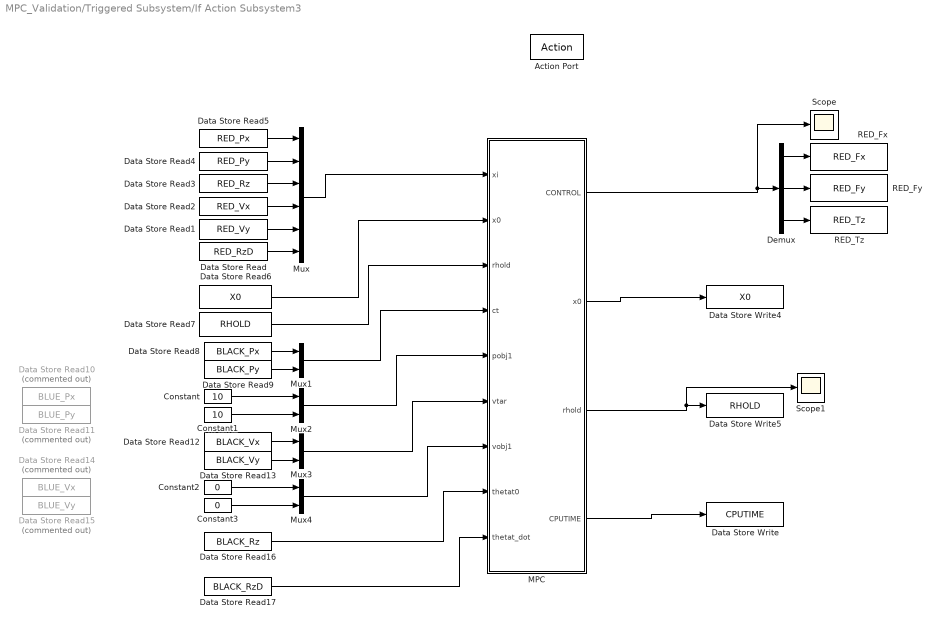
== system MPC_Validation/Triggered Subsystem/If Action Subsystem3 ==
  Action Port : ActionPort  ActionPortLabel=elseif(u1 == 5 & u2 == 1)
  Constant : Constant  Value=10
  Constant1 : Constant  Value=10
  Constant2 : Constant  Value=0
  Constant3 : Constant  Value=0
  Data Store Read : DataStoreRead  DataStoreName=RED_RzD
  Data Store Read1 : DataStoreRead  DataStoreName=RED_Vy
  Data Store Read10 : DataStoreRead  Commented=on  DataStoreName=BLUE_Px
  Data Store Read11 : DataStoreRead  Commented=on  DataStoreName=BLUE_Py
  Data Store Read12 : DataStoreRead  DataStoreName=BLACK_Vx
  Data Store Read13 : DataStoreRead  DataStoreName=BLACK_Vy
  Data Store Read14 : DataStoreRead  Commented=on  DataStoreName=BLUE_Vx
  Data Store Read15 : DataStoreRead  Commented=on  DataStoreName=BLUE_Vy
  Data Store Read16 : DataStoreRead  DataStoreName=BLACK_Rz
  Data Store Read17 : DataStoreRead  DataStoreName=BLACK_RzD
  Data Store Read2 : DataStoreRead  DataStoreName=RED_Vx
  Data Store Read3 : DataStoreRead  DataStoreName=RED_Rz
  Data Store Read4 : DataStoreRead  DataStoreName=RED_Py
  Data Store Read5 : DataStoreRead  DataStoreName=RED_Px
  Data Store Read6 : DataStoreRead  DataStoreName=X0
  Data Store Read7 : DataStoreRead  DataStoreName=RHOLD
  Data Store Read8 : DataStoreRead  DataStoreName=BLACK_Px
  Data Store Read9 : DataStoreRead  DataStoreName=BLACK_Py
  Data Store Write : DataStoreWrite  DataStoreName=CPUTIME
  Data Store Write4 : DataStoreWrite  DataStoreName=X0
  Data Store Write5 : DataStoreWrite  DataStoreName=RHOLD
  Demux : Demux  Outputs=3
  MPC : MATLAB Function  TreatAsAtomicUnit=on
  Mux : Mux  Inputs=6
  Mux{1..4} (4 alike) : Mux  Inputs=2
  RED_Fx : DataStoreWrite  DataStoreName=RED_Fx
  RED_Fy : DataStoreWrite  DataStoreName=RED_Fy
  RED_Tz : DataStoreWrite  DataStoreName=RED_Tz
  Scope : Scope
  Scope1 : Scope
  wires:
  Mux1/1 -> MPC/4(ct)
  Data Store Read17/1 -> MPC/9(thetat_dot)
  Data Store Read16/1 -> MPC/8(thetat0)
  Mux4/1 -> MPC/7(vobj1)
  Data Store Read6/1 -> MPC/2("x0 ")
  Data Store Read7/1 -> MPC/3("rhold ")
  Mux2/1 -> MPC/5(pobj1)
  Data Store Read12/1 -> Mux3/1
  Mux3/1 -> MPC/6(vtar)
  Data Store Read9/1 -> Mux1/2
  Data Store Read2/1 -> Mux/4
  MPC/2(x0) -> Data Store Write4/1
  MPC/3(rhold) -> Data Store Write5/1, Scope1/1
  Demux/2 -> RED_Fy/1
  Data Store Read/1 -> Mux/6
  MPC/1(CONTROL) -> Scope/1, Demux/1
  Demux/1 -> RED_Fx/1
  Demux/3 -> RED_Tz/1
  Mux/1 -> MPC/1(xi)
  Data Store Read1/1 -> Mux/5
  Data Store Read13/1 -> Mux3/2
  Data Store Read3/1 -> Mux/3
  Data Store Read5/1 -> Mux/1
  Data Store Read8/1 -> Mux1/1
  Data Store Read4/1 -> Mux/2
  MPC/4(CPUTIME) -> Data Store Write/1
  Constant/1 -> Mux2/1
  Constant1/1 -> Mux2/2
  Constant2/1 -> Mux4/1
  Constant3/1 -> Mux4/2

== system MPC_Validation/Triggered Subsystem/If Action Subsystem4 ==
  Action Port : ActionPort  ActionPortLabel=elseif( u1 == 6 & u2 == 1)
  Data Store Read : DataStoreRead  DataStoreName=RED_RzD
  Data Store Read1 : DataStoreRead  DataStoreName=RED_Vy
  Data Store Read10 : DataStoreRead  DataStoreName=BLUE_Px
  Data Store Read11 : DataStoreRead  DataStoreName=BLUE_Py
  Data Store Read12 : DataStoreRead  DataStoreName=BLACK_Vx
  Data Store Read13 : DataStoreRead  DataStoreName=BLACK_Vy
  Data Store Read14 : DataStoreRead  DataStoreName=BLUE_Vx
  Data Store Read15 : DataStoreRead  DataStoreName=BLUE_Vy
  Data Store Read16 : DataStoreRead  DataStoreName=BLACK_Rz
  Data Store Read17 : DataStoreRead  DataStoreName=BLACK_RzD
  Data Store Read2 : DataStoreRead  DataStoreName=RED_Vx
  Data Store Read3 : DataStoreRead  DataStoreName=RED_Rz
  Data Store Read4 : DataStoreRead  DataStoreName=RED_Py
  Data Store Read5 : DataStoreRead  DataStoreName=RED_Px
  Data Store Read6 : DataStoreRead  DataStoreName=X0
  Data Store Read7 : DataStoreRead  DataStoreName=RHOLD
  Data Store Read8 : DataStoreRead  DataStoreName=BLACK_Px
  Data Store Read9 : DataStoreRead  DataStoreName=BLACK_Py
  Data Store Write : DataStoreWrite  DataStoreName=CPUTIME
  Data Store Write4 : DataStoreWrite  DataStoreName=X0
  Data Store Write5 : DataStoreWrite  DataStoreName=RHOLD
  Demux : Demux  Outputs=3
  MPC : MATLAB Function  TreatAsAtomicUnit=on
  Mux : Mux  Inputs=6
  Mux{1..4} (4 alike) : Mux  Inputs=2
  RED_Fx : DataStoreWrite  DataStoreName=RED_Fx
  RED_Fy : DataStoreWrite  DataStoreName=RED_Fy
  RED_Tz : DataStoreWrite  DataStoreName=RED_Tz
  Scope : Scope
  Scope1 : Scope
  wires:
  MPC/4(CPUTIME) -> Data Store Write/1
  Data Store Read10/1 -> Mux2/1
  Data Store Read4/1 -> Mux/2
  Data Store Read14/1 -> Mux4/1
  Data Store Read8/1 -> Mux1/1
  Data Store Read5/1 -> Mux/1
  Data Store Read11/1 -> Mux2/2
  Data Store Read3/1 -> Mux/3
  Data Store Read13/1 -> Mux3/2
  Data Store Read1/1 -> Mux/5
  Mux/1 -> MPC/1(xi)
  Demux/3 -> RED_Tz/1
  Demux/1 -> RED_Fx/1
  MPC/1(CONTROL) -> Demux/1, Scope/1
  Data Store Read/1 -> Mux/6
  Demux/2 -> RED_Fy/1
  MPC/3(rhold) -> Scope1/1, Data Store Write5/1
  MPC/2(x0) -> Data Store Write4/1
  Data Store Read15/1 -> Mux4/2
  Data Store Read2/1 -> Mux/4
  Data Store Read9/1 -> Mux1/2
  Mux3/1 -> MPC/6(vtar)
  Data Store Read12/1 -> Mux3/1
  Mux2/1 -> MPC/5(pobj1)
  Data Store Read7/1 -> MPC/3("rhold ")
  Data Store Read6/1 -> MPC/2("x0 ")
  Mux4/1 -> MPC/7(vobj1)
  Data Store Read16/1 -> MPC/8(thetat0)
  Data Store Read17/1 -> MPC/9(thetat_dot)
  Mux1/1 -> MPC/4(ct)

== system MPC_Validation/Triggered Subsystem/If Action Subsystem5 ==
  Action Port : ActionPort  ActionPortLabel=elseif( u1 == 7 & u2 == 1)
  Data Store Read : DataStoreRead  DataStoreName=RED_RzD
  Data Store Read1 : DataStoreRead  DataStoreName=RED_Vy
  Data Store Read10 : DataStoreRead  DataStoreName=BLUE_Px
  Data Store Read11 : DataStoreRead  DataStoreName=BLUE_Py
  Data Store Read12 : DataStoreRead  DataStoreName=BLACK_Vx
  Data Store Read13 : DataStoreRead  DataStoreName=BLACK_Vy
  Data Store Read14 : DataStoreRead  DataStoreName=BLUE_Vx
  Data Store Read15 : DataStoreRead  DataStoreName=BLUE_Vy
  Data Store Read16 : DataStoreRead  DataStoreName=BLACK_Rz
  Data Store Read17 : DataStoreRead  DataStoreName=BLACK_RzD
  Data Store Read2 : DataStoreRead  DataStoreName=RED_Vx
  Data Store Read3 : DataStoreRead  DataStoreName=RED_Rz
  Data Store Read4 : DataStoreRead  DataStoreName=RED_Py
  Data Store Read5 : DataStoreRead  DataStoreName=RED_Px
  Data Store Read6 : DataStoreRead  DataStoreName=X0
  Data Store Read7 : DataStoreRead  DataStoreName=RHOLD
  Data Store Read8 : DataStoreRead  DataStoreName=BLACK_Px
  Data Store Read9 : DataStoreRead  DataStoreName=BLACK_Py
  Data Store Write : DataStoreWrite  DataStoreName=CPUTIME
  Data Store Write4 : DataStoreWrite  DataStoreName=X0
  Data Store Write5 : DataStoreWrite  DataStoreName=RHOLD
  Demux : Demux  Outputs=3
  MPC : MATLAB Function  TreatAsAtomicUnit=on
  Mux : Mux  Inputs=6
  Mux{1..4} (4 alike) : Mux  Inputs=2
  RED_Fx : DataStoreWrite  DataStoreName=RED_Fx
  RED_Fy : DataStoreWrite  DataStoreName=RED_Fy
  RED_Tz : DataStoreWrite  DataStoreName=RED_Tz
  Scope : Scope
  Scope1 : Scope
  wires:
  Mux1/1 -> MPC/4(ct)
  Data Store Read17/1 -> MPC/9(thetat_dot)
  Data Store Read16/1 -> MPC/8(thetat0)
  Mux4/1 -> MPC/7(vobj1)
  Data Store Read6/1 -> MPC/2("x0 ")
  Data Store Read7/1 -> MPC/3("rhold ")
  Mux2/1 -> MPC/5(pobj1)
  Data Store Read12/1 -> Mux3/1
  Mux3/1 -> MPC/6(vtar)
  Data Store Read9/1 -> Mux1/2
  Data Store Read2/1 -> Mux/4
  Data Store Read15/1 -> Mux4/2
  MPC/2(x0) -> Data Store Write4/1
  MPC/3(rhold) -> Data Store Write5/1, Scope1/1
  Demux/2 -> RED_Fy/1
  Data Store Read/1 -> Mux/6
  MPC/1(CONTROL) -> Scope/1, Demux/1
  Demux/1 -> RED_Fx/1
  Demux/3 -> RED_Tz/1
  Mux/1 -> MPC/1(xi)
  Data Store Read1/1 -> Mux/5
  Data Store Read13/1 -> Mux3/2
  Data Store Read3/1 -> Mux/3
  Data Store Read11/1 -> Mux2/2
  Data Store Read5/1 -> Mux/1
  Data Store Read8/1 -> Mux1/1
  Data Store Read14/1 -> Mux4/1
  Data Store Read4/1 -> Mux/2
  Data Store Read10/1 -> Mux2/1
  MPC/4(CPUTIME) -> Data Store Write/1

== system MPC_Validation/From Force//Torque to PWM Signal/Change BLACK Behavior/Calculate Thruster ON//OFF ==
  note: Calculate which thrusters must be turned on and for how long.
  note: The H matrix is not square, thus a pserudo-inverse is required.
  note: Knowing how much force each thruster can output, we can determine the saturated thruster output and then convert is into a percentage of time over which each thruster is open.
  note: After finding the PWM value, we can use the H matrix to go back to torque and force. However, these torques and forces will be "saturated".
  "[Fx_b; Fy_b; Tz]" : Inport
  BLACK_Fx_Sat : DataStoreWrite  DataStoreName=BLACK_Fx_Sat
  BLACK_Fy_Sat : DataStoreWrite  DataStoreName=BLACK_Fy_Sat
  BLACK_Rz : DataStoreRead  DataStoreName=BLACK_Rz
  BLACK_Tz_Sat : DataStoreWrite  DataStoreName=BLACK_Tz_Sat
  Data Store Write2 : DataStoreWrite  DataStoreName=BLACK_Thruster_ON_Count
  Demux : Demux  Outputs=3
  Demux1 : Demux  Outputs=2
  MATLAB Function : MATLAB Function  TreatAsAtomicUnit=on
  MATLAB Function1 : MATLAB Function  TreatAsAtomicUnit=on
  MATLAB Function10 : MATLAB Function  TreatAsAtomicUnit=on
  MATLAB Function11 : MATLAB Function  TreatAsAtomicUnit=on
  MATLAB Function2 : MATLAB Function  TreatAsAtomicUnit=on
  Mux : Mux  Inputs=2
  Product : Product  Multiplication=Matrix(*)
  Product1 : Product  Multiplication=Matrix(*)
  Product5 : Product  Multiplication=Matrix(*)
  Remove Negatives : Saturate  UpperLimit=1000  LowerLimit=0
  Rotate Forces to Inertial : Subsystem
  pseudo-inverse : Subsystem
  pseudo-inverse3 : Subsystem
  ThrusterPWM : Outport  VectorParamsAs1DForOutWhenUnconnected=off
  wires:
  pseudo-inverse/1(invH) -> Product/1
  "[Fx_b; Fy_b; Tz]"/1 -> Product5/2, Product/2
  MATLAB Function/1(H) -> pseudo-inverse/1(H)
  Remove Negatives/1 -> MATLAB Function2/1(ThrustPer)
  MATLAB Function1/1(H) -> Product1/1
  Product1/1 -> Demux/1
  Demux/2 -> Mux/2
  Demux/1 -> Mux/1
  Mux/1 -> Rotate Forces to Inertial/1("F_b ")
  BLACK_Rz/1 -> Rotate Forces to Inertial/2(Rz)
  Demux/3 -> BLACK_Tz_Sat/1
  Rotate Forces to Inertial/1(F_I) -> Demux1/1
  Demux1/1 -> BLACK_Fx_Sat/1
  Demux1/2 -> BLACK_Fy_Sat/1
  MATLAB Function2/1(ThrustPer_Final) -> Product1/2, ThrusterPWM/1
  Product/1 -> MATLAB Function10/1(PWMs)
  MATLAB Function10/2(count) -> Data Store Write2/1
  MATLAB Function10/1(thrust_decay_factor) -> MATLAB Function11/1(thrust_decay_factor)
  MATLAB Function11/1(H) -> pseudo-inverse3/1(H)
  pseudo-inverse3/1(invH) -> Product5/1
  Product5/1 -> Remove Negatives/1

== system MPC_Validation/From Force//Torque to PWM Signal/Change BLACK Behavior/Rotate Forces to Body ==
  "F_I " : Inport
  Rz : Inport  Port=2
  Create Rotation Matrix : MATLAB Function  TreatAsAtomicUnit=on
  Rotate F_I to F_b : Product  Multiplication=Matrix(*)
  F_b : Outport  VectorParamsAs1DForOutWhenUnconnected=off
  wires:
  Rotate F_I to F_b/1 -> F_b/1
  Create Rotation Matrix/1(C_bI) -> Rotate F_I to F_b/1
  "F_I "/1 -> Rotate F_I to F_b/2
  Rz/1 -> Create Rotation Matrix/1(Rz)

== system MPC_Validation/From Force//Torque to PWM Signal/Change BLUE Behavior/Calculate Thruster ON//OFF ==
  note: Calculate which thrusters must be turned on and for how long.
  note: The H matrix is not square, thus a pserudo-inverse is required.
  note: Knowing how much force each thruster can output, we can determine the saturated thruster output and then convert is into a percentage of time over which each thruster is open.
  note: After finding the PWM value, we can use the H matrix to go back to torque and force. However, these torques and forces will be "saturated".
  "[Fx_b; Fy_b; Tz]" : Inport
  BLUE_Fx_Sat : DataStoreWrite  DataStoreName=BLUE_Fx_Sat
  BLUE_Fy_Sat : DataStoreWrite  DataStoreName=BLUE_Fy_Sat
  BLUE_Rz : DataStoreRead  DataStoreName=BLUE_Rz
  BLUE_Tz_Sat : DataStoreWrite  DataStoreName=BLUE_Tz_Sat
  Data Store Write1 : DataStoreWrite  DataStoreName=BLUE_Thruster_ON_Count
  Demux : Demux  Outputs=3
  Demux1 : Demux  Outputs=2
  MATLAB Function : MATLAB Function  TreatAsAtomicUnit=on
  MATLAB Function1 : MATLAB Function  TreatAsAtomicUnit=on
  MATLAB Function2 : MATLAB Function  TreatAsAtomicUnit=on
  MATLAB Function6 : MATLAB Function  TreatAsAtomicUnit=on
  MATLAB Function7 : MATLAB Function  TreatAsAtomicUnit=on
  Mux : Mux  Inputs=2
  Product : Product  Multiplication=Matrix(*)
  Product1 : Product  Multiplication=Matrix(*)
  Product4 : Product  Multiplication=Matrix(*)
  Remove Negatives : Saturate  UpperLimit=1000  LowerLimit=0
  Rotate Forces to Inertial : Subsystem
  pseudo-inverse : Subsystem
  pseudo-inverse2 : Subsystem
  ThrusterPWM : Outport  VectorParamsAs1DForOutWhenUnconnected=off
  wires:
  pseudo-inverse/1(invH) -> Product/1
  MATLAB Function/1(H) -> pseudo-inverse/1(H)
  Remove Negatives/1 -> MATLAB Function2/1(ThrustPer)
  MATLAB Function1/1(H) -> Product1/1
  Product1/1 -> Demux/1
  Demux/2 -> Mux/2
  Demux/1 -> Mux/1
  Mux/1 -> Rotate Forces to Inertial/1("F_b ")
  BLUE_Rz/1 -> Rotate Forces to Inertial/2(Rz)
  Demux/3 -> BLUE_Tz_Sat/1
  Rotate Forces to Inertial/1(F_I) -> Demux1/1
  Demux1/1 -> BLUE_Fx_Sat/1
  Demux1/2 -> BLUE_Fy_Sat/1
  MATLAB Function2/1(ThrustPer_Final) -> Product1/2, ThrusterPWM/1
  MATLAB Function6/2(count) -> Data Store Write1/1
  pseudo-inverse2/1(invH) -> Product4/1
  Product/1 -> MATLAB Function6/1(PWMs)
  MATLAB Function6/1(thrust_decay_factor) -> MATLAB Function7/1(thrust_decay_factor)
  MATLAB Function7/1(H) -> pseudo-inverse2/1(H)
  "[Fx_b; Fy_b; Tz]"/1 -> Product4/2, Product/2
  Product4/1 -> Remove Negatives/1

== system MPC_Validation/From Force//Torque to PWM Signal/Change BLUE Behavior/Rotate Forces to Body ==
  "F_I " : Inport
  Rz : Inport  Port=2
  Create Rotation Matrix : MATLAB Function  TreatAsAtomicUnit=on
  Rotate F_I to F_b : Product  Multiplication=Matrix(*)
  F_b : Outport  VectorParamsAs1DForOutWhenUnconnected=off
  wires:
  Rotate F_I to F_b/1 -> F_b/1
  Create Rotation Matrix/1(C_bI) -> Rotate F_I to F_b/1
  "F_I "/1 -> Rotate F_I to F_b/2
  Rz/1 -> Create Rotation Matrix/1(Rz)
